simulink model "NewtonsMethodonRiemannManifold"  (R2019a)
settings: Solver=VariableStepAuto  StartTime=0.0  StopTime=10.0  RelTol=1e-3
libraries: vrlib x4, dspstat3 x1
settings Model: Creator=Owner  LastModifiedBy=Owner

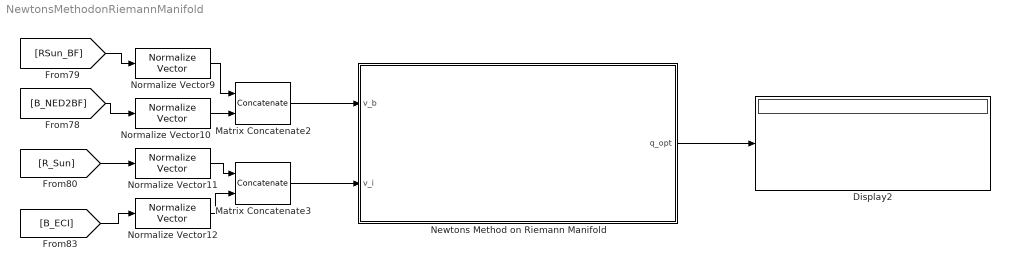
== system NewtonsMethodonRiemannManifold ==
  Display2 : Display
  Matrix Concatenate2 : Concatenate  Mode=Multidimensional array  ConcatenateDimension=2
  Matrix Concatenate3 : Concatenate  Mode=Multidimensional array  ConcatenateDimension=2
  Newtons Method on Riemann Manifold : Subsystem
  Normalize Vector{9..12} (4 alike) : vrlib/Utilities/Normalize Vector  maxzero=0
      settings: SourceProductName=Simulink
  wires:
  Normalize Vector9/1 -> Matrix Concatenate2/1
  Matrix Concatenate3/1 -> Newtons Method on Riemann Manifold/2(v_i)
  Matrix Concatenate2/1 -> Newtons Method on Riemann Manifold/1(v_b)
  Normalize Vector11/1 -> Matrix Concatenate3/1
  Normalize Vector10/1 -> Matrix Concatenate2/2
  Newtons Method on Riemann Manifold/1(q_opt) -> Display2/1
  [RSun_BF] -> Normalize Vector9/1
  [B_NED2BF] -> Normalize Vector10/1
  [B_ECI] -> Normalize Vector12/1
  [R_Sun] -> Normalize Vector11/1
  Normalize Vector12/1 -> Matrix Concatenate3/2

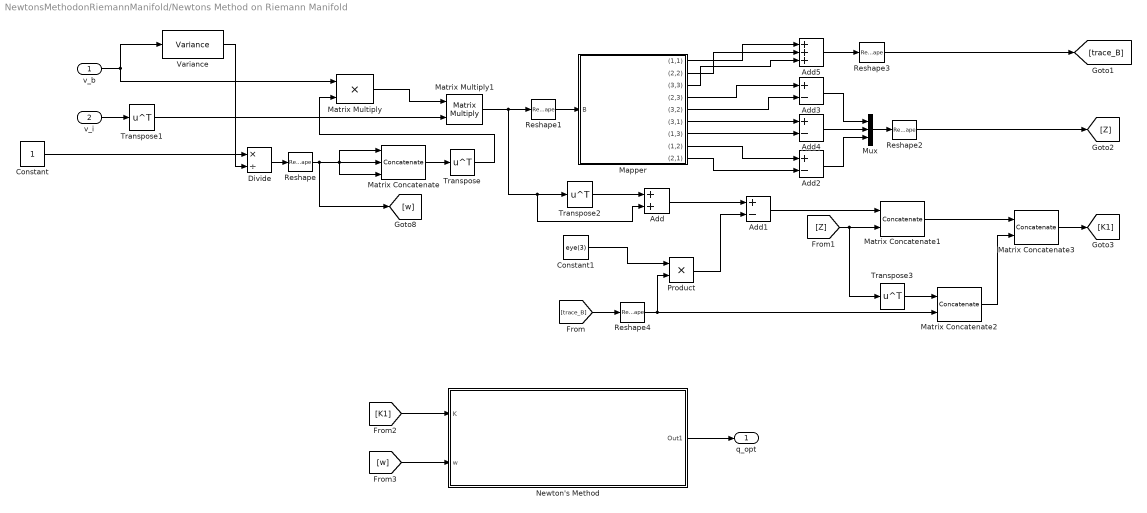
== system NewtonsMethodonRiemannManifold/Newtons Method on Riemann Manifold ==
  v_b : Inport
  v_i : Inport  Port=2
  Add : Sum
  Add{1..4} (4 alike) : Sum  Inputs=+-
  Add5 : Sum  Inputs=+++
  Constant : Constant
  Constant1 : Constant  Value=eye(3)
  Divide : Product  Inputs=*/
  Mapper : Subsystem
  Matrix Concatenate : Concatenate  NumInputs=3  Mode=Multidimensional array  ConcatenateDimension=2
  Matrix Concatenate1 : Concatenate  Mode=Multidimensional array  ConcatenateDimension=2
  Matrix Concatenate2 : Concatenate  Mode=Multidimensional array  ConcatenateDimension=2
  Matrix Concatenate3 : Concatenate  Mode=Multidimensional array
  Matrix Multiply : Product
  Matrix Multiply1 : Product  Multiplication=Matrix(*)
  Mux : Mux  Inputs=3
  Newton's Method : Subsystem
  Product : Product
  Reshape{,1..4} (5 alike) : Reshape  OutputDimensionality=Column vector (2-D)
  Transpose{,1..3} (4 alike) : Math  Operator=transpose  SaturateOnIntegerOverflow=on
  Variance : dspstat3/Variance  run=off  InputProcessing=Columns as channels (frame based)  reset_popup=None  directionMode=Each column  dimension=1  roiEnable=off  roiType=Rectangles  roiPortion=Entire ROI  roiOutput=Individual statistics for each ROI  roiFlag=off  roundingMode=Floor  overflowMode=off
      settings: SourceProductName=DSP System Toolbox
  q_opt : Outport
  wires:
  Reshape/1 -> [w], Matrix Concatenate/3, Matrix Concatenate/2, Matrix Concatenate/1
  Matrix Concatenate/1 -> Transpose/1
  Constant/1 -> Divide/1
  Variance/1 -> Divide/2
  v_i/1 -> Transpose1/1
  Matrix Multiply/1 -> Matrix Multiply1/1
  Transpose1/1 -> Matrix Multiply1/2
  Divide/1 -> Reshape/1
  Transpose/1 -> Matrix Multiply/2
  v_b/1 -> Matrix Multiply/1, Variance/1
  Matrix Multiply1/1 -> Add/2, Transpose2/1, Reshape1/1
  Mux/1 -> Reshape2/1
  Add3/1 -> Mux/1
  Mapper/9((2,1)) -> Add2/2
  Mapper/4((2,3)) -> Add3/1
  Reshape2/1 -> [Z]
  Add2/1 -> Mux/3
  Mapper/7((1,3)) -> Add4/2
  Add4/1 -> Mux/2
  Mapper/8((1,2)) -> Add2/1
  Mapper/5((3,2)) -> Add3/2
  Mapper/6((3,1)) -> Add4/1
  Transpose2/1 -> Add/1
  Reshape1/1 -> Mapper/1(B)
  Add/1 -> Add1/1
  Mapper/1((1,1)) -> Add5/1
  Mapper/2((2,2)) -> Add5/2
  Mapper/3((3,3)) -> Add5/3
  Add5/1 -> Reshape3/1
  Reshape3/1 -> [trace_B]
  [trace_B] -> Reshape4/1
  Constant1/1 -> Product/1
  Product/1 -> Add1/2
  Add1/1 -> Matrix Concatenate1/1
  [Z] -> Transpose3/1, Matrix Concatenate1/2
  Reshape4/1 -> Matrix Concatenate2/2, Product/2
  Transpose3/1 -> Matrix Concatenate2/1
  Matrix Concatenate1/1 -> Matrix Concatenate3/1
  Matrix Concatenate2/1 -> Matrix Concatenate3/2
  Matrix Concatenate3/1 -> [K1]
  [w] -> Newton's Method/2(w)
  [K1] -> Newton's Method/1(K)
  Newton's Method/1(Out1) -> q_opt/1

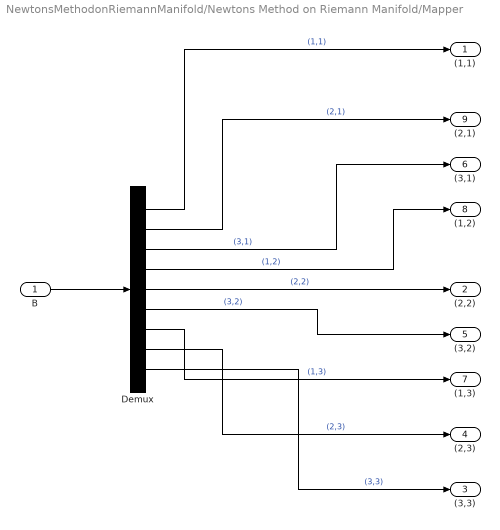
== system NewtonsMethodonRiemannManifold/Newtons Method on Riemann Manifold/Mapper ==
  B : Inport
  Demux : Demux  Outputs=9
  (1,1) : Outport
  (2,2) : Outport  Port=2
  (3,3) : Outport  Port=3
  (2,3) : Outport  Port=4
  (3,2) : Outport  Port=5
  (3,1) : Outport  Port=6
  (1,3) : Outport  Port=7
  (1,2) : Outport  Port=8
  (2,1) : Outport  Port=9
  wires:
  Demux/1 -> (1,1)/1  "(1,1)"
  Demux/7 -> (1,3)/1  "(1,3)"
  Demux/6 -> (3,2)/1  "(3,2)"
  Demux/5 -> (2,2)/1  "(2,2)"
  B/1 -> Demux/1
  Demux/3 -> (3,1)/1  "(3,1)"
  Demux/8 -> (2,3)/1  "(2,3)"
  Demux/9 -> (3,3)/1  "(3,3)"
  Demux/2 -> (2,1)/1  "(2,1)"
  Demux/4 -> (1,2)/1  "(1,2)"

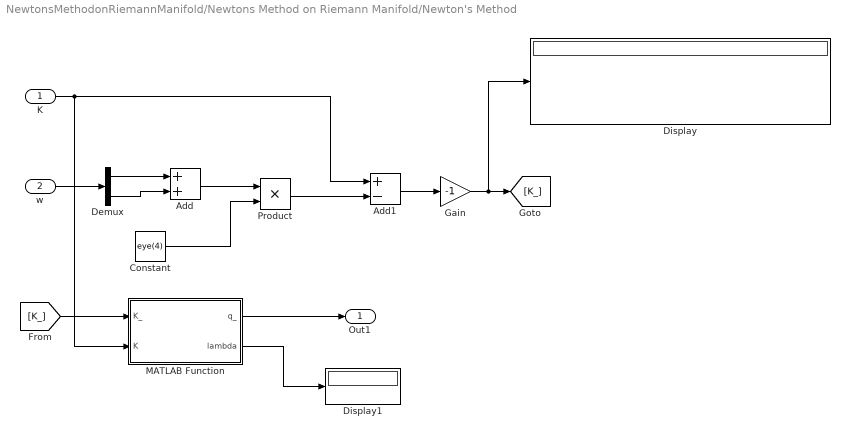
== system NewtonsMethodonRiemannManifold/Newtons Method on Riemann Manifold/Newton's Method ==
  K : Inport
  w : Inport  Port=2
  Add : Sum
  Add1 : Sum  Inputs=+-
  Constant : Constant  Value=eye(4)
  Demux : Demux  Outputs=2
  Display : Display
  Display1 : Display
  Gain : Gain  Gain=-1
  MATLAB Function : MATLAB Function  TreatAsAtomicUnit=on
  Product : Product
  Out1 : Outport
  wires:
  w/1 -> Demux/1
  Demux/1 -> Add/1
  Demux/2 -> Add/2
  Add/1 -> Product/1
  Constant/1 -> Product/2
  Product/1 -> Add1/2
  K/1 -> MATLAB Function/2(K), Add1/1
  Add1/1 -> Gain/1
  Gain/1 -> Display/1, [K_]
  [K_] -> MATLAB Function/1(K_)
  MATLAB Function/2(lambda) -> Display1/1
  MATLAB Function/1(q_) -> Out1/1

== matlab function NewtonsMethodonRiemannManifold/Newtons Method on Riemann Manifold/Newton's Method/MATLAB Function ==
  data: K_ input; q_ output; lambda output; K input
function [q_,lambda] = eig(K_,K)
q  = - K_(:,1:3)\K_(:,4);
q_ = [q; 1]/norm([q; 1]); % Initial eigenvector
lambda = q_'*K*q_; % Initial eigenvalue

while norm(K*q_- lambda*q_) > 10e-15 % K*q_opt = lambda_max*q_opt
    P_q = eye(4) - q_*q_';
    y   = [(P_q*K*P_q - q_'*K*q_*eye(4)); q_']\[- P_q*K*q_; 0]; % Eqn 6
    q_  = (q_ + y)/norm(q_ + y); % Eqn 7
    lambda = q_'*K*q_; % Eqn 2
end 
end
